simulink model "test1"  (R2014b)
settings: Solver=ode45  StartTime=0.0  StopTime=10.0  RelTol=1e-3
libraries: fuzblock x1
settings Model: Creator=Administrator  LastModifiedBy=Administrator
settings DebuggingCC: MaxConsecutiveZCsMsg=none

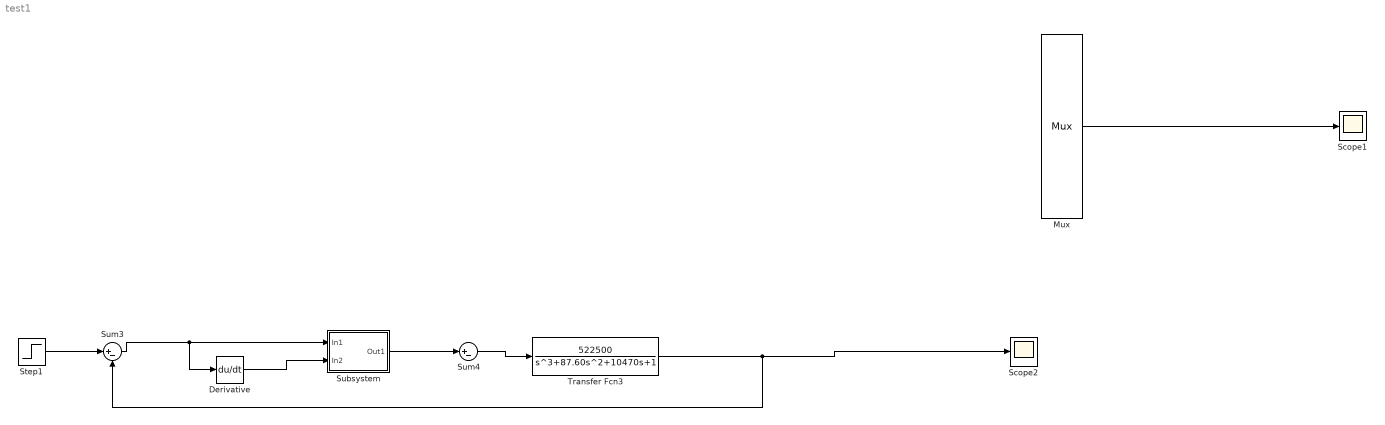
== system test1 ==
  Derivative : Derivative
  Mux : Mux  Inputs=2
  Scope1 : Scope
      settings: YMin=-1  YMax=1
  Scope2 : Scope
      settings: YMin=-1  YMax=1
  Step1 : Step  After=50  SampleTime=0
  Subsystem : Subsystem
  Sum3 : Sum  Inputs=|+-
  Sum4 : Sum  Inputs=|+-
  Transfer Fcn3 : TransferFcn  Numerator=[522500]  Denominator=[1 87.60 10470 1]
  wires:
  Step1/1 -> Sum3/1
  Sum4/1 -> Transfer Fcn3/1
  Sum3/1 -> Derivative/1, Subsystem/1(In1)
  Derivative/1 -> Subsystem/2(In2)
  Subsystem/1(Out1) -> Sum4/1
  Mux/1 -> Scope1/1
  Transfer Fcn3/1 -> Sum3/2, Scope2/1

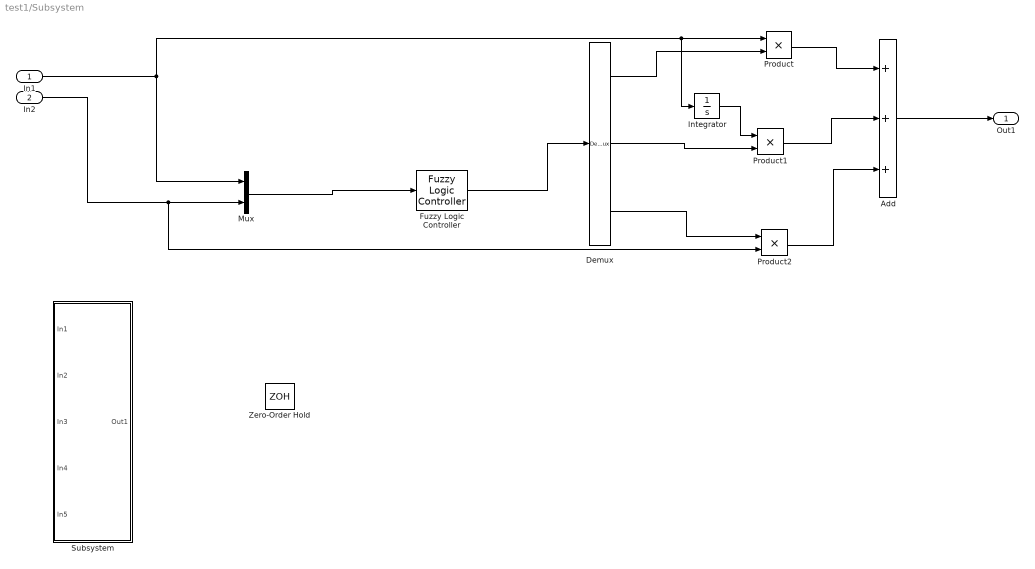
== system test1/Subsystem ==
  In1 : Inport
  In2 : Inport  Port=2
  Add : Sum  Inputs=+++
  Demux : Demux  Outputs=3
  Fuzzy Logic Controller : fuzblock/Fuzzy Logic  Controller  fis=fuzzy_y
  Integrator : Integrator
  Mux : Mux  Inputs=2
  Product : Product
  Product1 : Product
  Product2 : Product
  Subsystem : Subsystem
  Zero-Order Hold : ZeroOrderHold
  Out1 : Outport
  wires:
  In1/1 -> Mux/1, Integrator/1, Product/1
  In2/1 -> Product2/2, Mux/2
  Fuzzy Logic Controller/1 -> Demux/1
  Demux/3 -> Product2/1
  Demux/1 -> Product/2
  Integrator/1 -> Product1/1
  Demux/2 -> Product1/2
  Product/1 -> Add/1
  Product1/1 -> Add/2
  Product2/1 -> Add/3
  Add/1 -> Out1/1
  Mux/1 -> Fuzzy Logic Controller/1

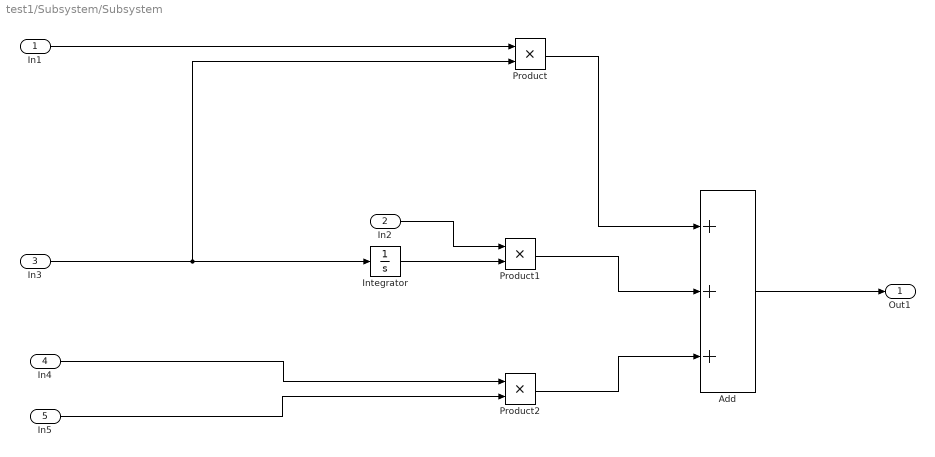
== system test1/Subsystem/Subsystem ==
  In1 : Inport
  In2 : Inport  Port=2
  In3 : Inport  Port=3
  In4 : Inport  Port=4
  In5 : Inport  Port=5
  Add : Sum  Inputs=+++
  Integrator : Integrator
  Product : Product
  Product1 : Product
  Product2 : Product
  Out1 : Outport
  wires:
  Product/1 -> Add/1
  In1/1 -> Product/1
  In2/1 -> Product1/1
  Product1/1 -> Add/2
  Product2/1 -> Add/3
  Integrator/1 -> Product1/2
  In3/1 -> Product/2, Integrator/1
  In4/1 -> Product2/1
  In5/1 -> Product2/2
  Add/1 -> Out1/1
